simulink model "mdl_7_1"  (R2024b)
settings: Solver=FixedStepAuto  StartTime=0.0  StopTime=300  FixedStep=1e-2  RelTol=1e-3
values from neighbouring files (symbols this model uses):
  Cd = diag([kd kd kd])    [init_7_1.m]
  J1 = [10000    0     0 ... (first row only)    [init_7_1.m]
  kp = 50    [init_7_1.m]
  q0 = [0.6853 0.6953 0.1531 0.1531]'    [init_7_1.m]
  w0 = [deg2rad(0.5300) deg2rad(0.5300) deg2rad(0.05300)]'    [init_7_1.m]
settings Model: Creator=Monster  LastModifiedBy=Monster

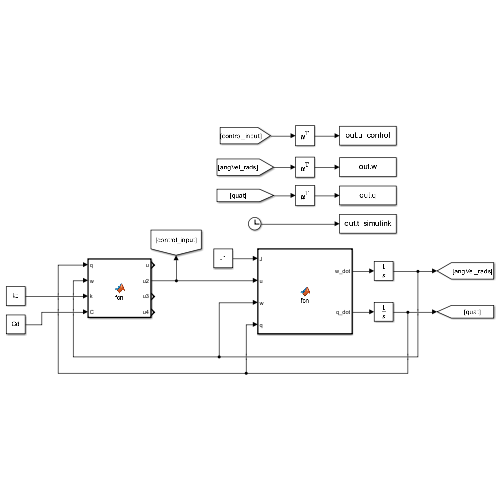
[thumbnail: Simulink's stored preview of the top-level diagram]
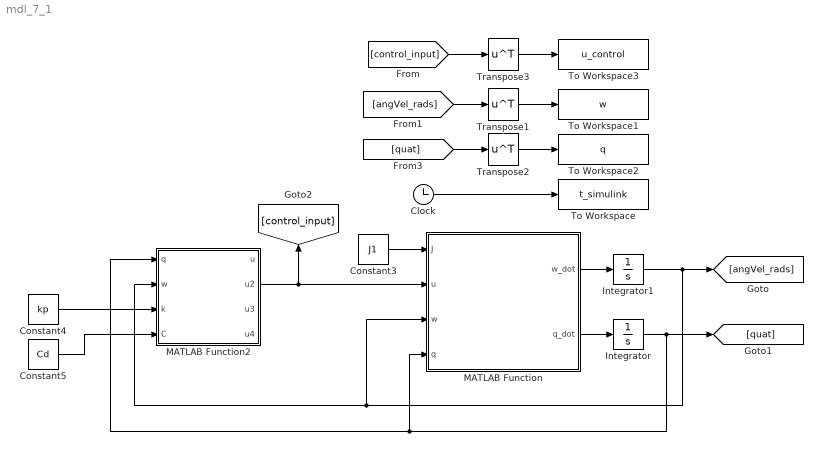
== system mdl_7_1 ==
  Clock : Clock
  Constant3 : Constant  Value=J1
  Constant4 : Constant  Value=kp
  Constant5 : Constant  Value=Cd
  Integrator : Integrator  InitialCondition=q0
  Integrator1 : Integrator  InitialCondition=w0
  MATLAB Function : MATLAB Function  TreatAsAtomicUnit=on
  MATLAB Function2 : MATLAB Function  TreatAsAtomicUnit=on
  To Workspace : ToWorkspace  VariableName=t_simulink  SampleTime=-1
      settings: Save2DSignal=2-D array (concatenate along first dimension)
  To Workspace1 : ToWorkspace  VariableName=w  SampleTime=-1
      settings: Save2DSignal=2-D array (concatenate along first dimension)
  To Workspace2 : ToWorkspace  VariableName=q  SampleTime=-1
      settings: Save2DSignal=2-D array (concatenate along first dimension)
  To Workspace3 : ToWorkspace  VariableName=u_control  SampleTime=-1
      settings: Save2DSignal=2-D array (concatenate along first dimension)
  Transpose1 : Math  Operator=transpose
  Transpose2 : Math  Operator=transpose
  Transpose3 : Math  Operator=transpose
  wires:
  Integrator/1 -> [quat], MATLAB Function2/1(q), MATLAB Function/4(q)
  Clock/1 -> To Workspace/1
  [quat] -> Transpose2/1
  Integrator1/1 -> [angVel_rads], MATLAB Function2/2(w), MATLAB Function/3(w)
  [angVel_rads] -> Transpose1/1
  MATLAB Function/2(q_dot) -> Integrator/1
  Transpose2/1 -> To Workspace2/1
  Transpose1/1 -> To Workspace1/1
  Constant3/1 -> MATLAB Function/1(J)
  MATLAB Function/1(w_dot) -> Integrator1/1
  Constant4/1 -> MATLAB Function2/3(k)
  Constant5/1 -> MATLAB Function2/4(C)
  MATLAB Function2/2(u2) -> MATLAB Function/2(u), [control_input]
  [control_input] -> Transpose3/1
  Transpose3/1 -> To Workspace3/1

== matlab function mdl_7_1/MATLAB Function ==
  data: w_dot output; J input; u input; q_dot output; w input; q input
function [w_dot,q_dot] = fcn(J,u,w,q)


w1 = w(1);
w2 = w(2);
w3 = w(3);

W = [ 0,  w3, -w2, w1;
    -w3,   0,  w1, w2;
     w2, -w1,   0, w3;
    -w1, -w2, -w3,  0 ];

% output
w_dot = inv(J)*(u-cross(w,J*w));

q_dot = 0.5*W*q;

end

== matlab function mdl_7_1/MATLAB Function2 ==
  data: u output; u2 output; q input; w input; k input; C input; u3 output; u4 output
function [u,u2,u3,u4]= fcn(q,w,k,C)

I3x3 = eye(3,3);
K = k*I3x3;

% Controller I
% Controller II
K2 = k*sign(q(4))*I3x3;
% Controller III
C3 = C*(1+transpose(q(1:3))*q(1:3));
% Controller IIII
C4 = C*(1-transpose(q(1:3))*q(1:3));

u  = -K*q(1:3) - C*w;
u2 = -K2*q(1:3) - C*w;
u3 = -K2*q(1:3) - C3*w;
u4 = -K2*q(1:3) - C4*w;

end
